simulink model "rtwdemo_mdlreftop"  (Simulink 7.6)
settings: Solver=FixedStepDiscrete  SolverMode=SingleTasking  StartTime=0.0  StopTime=10.0  FixedStep=0.1  RelTol=1e-3
Description:
  | File Packaging for Models (Code and Data)
settings Model: Creator=The MathWorks Inc.  ExtModeAutoUpdateStatusClock=off
settings MATStruct: SampleTime=0.1  Offset=0  Priority=[20.0]
settings DataIOCC: LimitDataPoints=off  SaveFormat=StructureWithTime  SaveOutput=off  SaveTime=off  SignalLoggingName=logsOut
settings OptimizationCC: InlineParams=on  InlineInvariantSignals=on  StateBitsets=on  DataBitsets=on  UseTempVars=on  EfficientFloat2IntCast=on  EfficientMapNaN2IntZero=off
settings DebuggingCC: CheckExecutionContextPreStartOutputMsg=on  CheckExecutionContextRuntimeOutputMsg=on  SolverPrmCheckMsg=none  StrictBusMsg=ErrorOnBusTreatedAsVector
settings HardwareCC: ProdIntDivRoundTo=Zero  ProdEndianess=LittleEndian  ProdHWDeviceType=Generic->32-bit Embedded Processor  TargetHWDeviceType=Generic->32-bit Embedded Processor
settings ModelReferenceCC: UpdateModelReferenceTargets=IfOutOfDate  CheckModelReferenceTargetMessage=none
settings RTWCC: TLCOptions=-p0 -aWarnNonSaturatedBlocks=0  GenerateReport=on  RTWVerbose=off  ProcessScript=grt_make_rtw_hook  LaunchReport=on
settings CodeAppCC: ForceParamTrailComments=on  MaxIdLength=128
settings GRTTargetCC: TargetFcnLib=ansi_tfl_tmw.mat

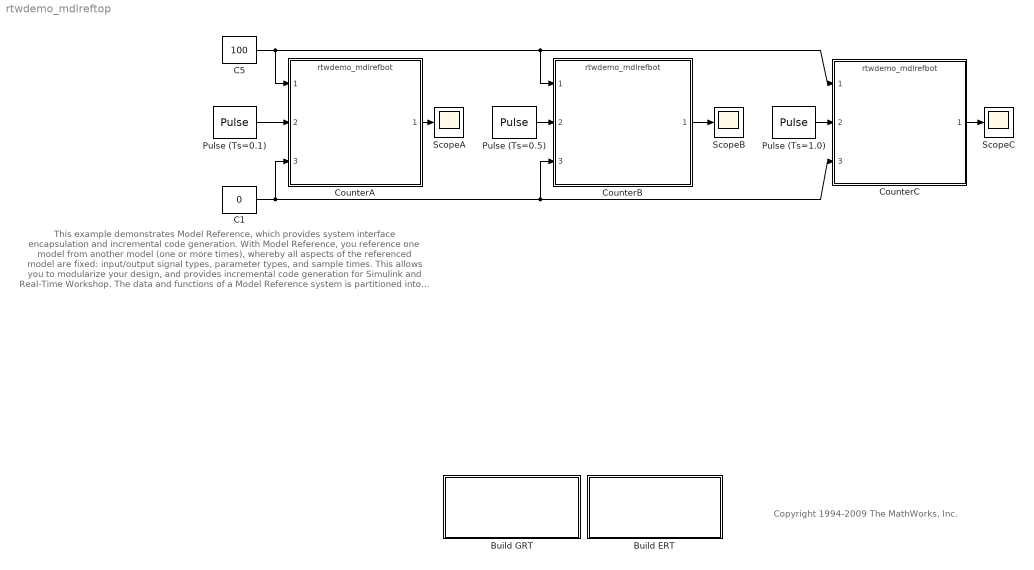
== system rtwdemo_mdlreftop ==
  note: This example demonstrates Model Reference, which provides system interface encapsulation and incremental code generation.
      | With Model Reference, you reference one model from another model (one or more times), whereby all aspects of the referenced
      | model are fixed: input/output signal types, parameter types, and sample times.  This allows you to modularize your
      | design, and provides incremental code generation for Simulink and Real-Time Workshop.
      |
      | The data and functions of a Model Reference system is partitioned into its own set of files, independent of its parent
      | model. In this example, the model rtwdemo_mdlrefbot.mdl is referenced three times.  For simulation and code generation,
      | the model is incrementally generated.  That is, rtwdemo_mdlrefbot.mdl will build the first time, but not on subsequent
      | builds (until rtwdemo_mdlrefbot.mdl is changed).
      |
      | Since Model Reference shares and manages code for models, each RTW target must be built into its own directory.  The
      | blue buttons below generate code for Real-Time Workshop and Real-Time Workshop Embedded Coder.
  note: Copyright 1994-2009 The MathWorks, Inc.
  Build ERT : Subsystem  mask{attrib_overrides=}
      mask prompts: attrib_overrides "List of attributes to preserve (cell of strings):"
      mask help: Enter the attributes of the configuration set that you want preserved. Otherwise, the default configuration script will override your current settings.
      settings: OpenFcn=|
      | if ~exist('rtwdemo_ert', 'dir')
      |     disp('Creating working directory rtwdemo_ert')
      |     mkdir('rtwdemo_ert')
      | end
      | cd('rtwdemo_ert');
      | overrides=get_param(gcb,'attrib_overrides');
      | modelbot='rtwdemo_mdlrefbot';
      | load_system(modelbot);
      | ori_cs_bot = getActiveConfigSet(modelbot);
      | tmp_cs_bot = ori_cs_bot.copy;
      | tmp_cs_bot.Name = 'tempcs4bot';
      | attachConfigSet(modelbot, tmp_cs_bot);
      | setActiveConfigSet(modelbot, 'tempcs4bot');
      | rtwconfiguredemo(modelbot,'noop',false,overrides);
      | setProp(tmp_cs_bot,'CustomSymbolStr','$R$N$M');
      | set_param(modelbot,'dirty','off');
      | 
      | modeltop='rtwdemo_mdlreftop';
      | ori_cs_top=getActiveConfigSet(modeltop);
      | tmp_cs_top = ori_cs_top.copy;
      | tmp_cs_top.Name = 'tempcs4top';
      | attachConfigSet(modeltop, tmp_cs_top);
      | setActiveConfigSet(modeltop, 'tempcs4top');
      | 
      | rtwconfiguredemo(modeltop,'noop',false,overrides);
      | setProp(tmp_cs_top,'CustomSymbolStr','$R$N$M');
      | 
      | rtwbuilddemomodel(modeltop);
      | cd('..')
      | 
      | setActiveConfigSet(modelbot, ori_cs_bot.Name);
      | setActiveConfigSet(modeltop, ori_cs_top.Name);
      | tmp_cs_bot = detachConfigSet(modelbot, tmp_cs_bot.Name);
      | tmp_cs_top = detachConfigSet(modeltop, tmp_cs_top.Name);
      | 
      | set_param(modeltop,'dirty','off');
      | set_param(modelbot,'dirty','off');
      | close_system(modelbot);
      | 
      | clear modeltop modelbot overrides ori_cs_bot ori_cs_top tmp_cs_bot tmp_cs_top;
      mask Display:
      | disp(['Generate Code Using\n',...
      | 	  'Real-Time Workshop\n',...
      | 	  'Embedded Coder\n'...
      | 	  '(double-click)'])
  Build GRT : Subsystem  mask{attrib_overrides={}}
      mask prompts: attrib_overrides "List of attributes to preserve (cell of strings):"
      mask help: Enter the attributes of the configuration set that you want preserved. Otherwise, the default configuration script will override your current settings.
      settings: OpenFcn=|
      | try
      |   if ~exist('rtwdemo_grt','dir')
      |     disp('Creating working directory rtwdemo_grt')
      |     mkdir('rtwdemo_grt');
      |   end
      |   chdir('rtwdemo_grt')
      |   overrides=get_param(gcb,'attrib_overrides');
      |   model='rtwdemo_mdlrefbot';
      |   load_system(model);
      |   rtwconfiguredemo(model,'noop',true,overrides);
      |   model='rtwdemo_mdlreftop';
      |   rtwconfiguredemo(model,'noop',true,overrides);
      |   rtwbuilddemomodel(model);
      |   cd('..');
      | catch
      |   error(lasterr);
      | end
      | 
      |  clear model overrides;
      mask Display:
      | disp(['Generate Code Using\n',...
      | 	  'Real-Time Workshop\n',...
      | 	  '(double-click)'])
  C1 : Constant  Value=0
  C5 : Constant  Value=100
  CounterA : ModelReference  ModelNameDialog=rtwdemo_mdlrefbot  SimulationMode=Accelerator  ModelReferenceVersion=1.82  CopyOfModelName=rtwdemo_mdlrefbot
  CounterB : ModelReference  ModelNameDialog=rtwdemo_mdlrefbot  SimulationMode=Accelerator  ModelReferenceVersion=1.82  CopyOfModelName=rtwdemo_mdlrefbot
  CounterC : ModelReference  ModelNameDialog=rtwdemo_mdlrefbot  SimulationMode=Accelerator  ModelReferenceVersion=1.82  CopyOfModelName=rtwdemo_mdlrefbot
  Pulse (Ts=0.1) : DiscretePulseGenerator  SampleTime=0.1  VectorParams1D=off
  Pulse (Ts=0.5) : DiscretePulseGenerator  SampleTime=0.5
  Pulse (Ts=1.0) : DiscretePulseGenerator  SampleTime=1.0
  ScopeA : Scope
      settings: TimeRange=10  YMin=0  YMax=100
  ScopeB : Scope
      settings: TimeRange=10  YMin=0  YMax=25
  ScopeC : Scope
      settings: TimeRange=10  YMin=0  YMax=15  SaveName=ScopeData2
  wires:
  CounterB/1 -> ScopeB/1
  CounterA/1 -> ScopeA/1
  CounterC/1 -> ScopeC/1
  Pulse (Ts=0.1)/1 -> CounterA/2
  Pulse (Ts=0.5)/1 -> CounterB/2
  Pulse (Ts=1.0)/1 -> CounterC/2
  C1/1 -> CounterC/3, CounterB/3, CounterA/3
  C5/1 -> CounterA/1, CounterB/1, CounterC/1

== system rtwdemo_mdlreftop/Build ERT ==

== system rtwdemo_mdlreftop/Build GRT ==
